simulink model "CP_DTSFC_Lin_b_9558292"  (R2018a)
settings: Solver=FixedStepDiscrete  StartTime=0.0  StopTime=3  FixedStep=T_s  RelTol=1e-3
values from neighbouring files (symbols this model uses):
  K_db = place(sysdzoh.A,sysdzoh.B,Pb_d)    [CP_DTSFC_Lin_b_MainFile_9558292.m]
  sysdzoh = c2d(sysc,T_s,'zoh')    [CP_DTSFC_Lin_a_MainFile_n9558292.m]    (also in CP_DTSFC_Lin_b_MainFile_9558292.m)
  T_s = 0.03    [CP_DTSFC_Lin_a_MainFile_n9558292.m]    (also in CP_DTSFC_Lin_b_MainFile_9558292.m)
  x10 = 0.2    [CP_DTSFC_Lin_a_MainFile_n9558292.m]    (also in CP_DTSFC_Lin_b_MainFile_9558292.m)
  x20 = deg2rad(20)    [CP_DTSFC_Lin_a_MainFile_n9558292.m]    (also in CP_DTSFC_Lin_b_MainFile_9558292.m)
  x30 = 0    [CP_DTSFC_Lin_a_MainFile_n9558292.m]    (also in CP_DTSFC_Lin_b_MainFile_9558292.m)
  x40 = 0    [CP_DTSFC_Lin_a_MainFile_n9558292.m]    (also in CP_DTSFC_Lin_b_MainFile_9558292.m)
settings Model: Creator=haidarobeid  LastModifiedBy=haidarobeid

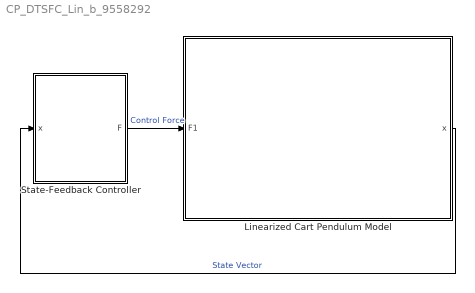
== system CP_DTSFC_Lin_b_9558292 ==
  Linearized Cart Pendulum Model : Subsystem
  State-Feedback Controller : Subsystem
  wires:
  Linearized Cart Pendulum Model/1(x) -> State-Feedback Controller/1(x)  "State Vector"
  State-Feedback Controller/1(F) -> Linearized Cart Pendulum Model/1(F1)  "Control Force"

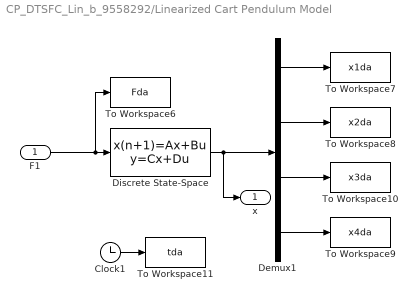
== system CP_DTSFC_Lin_b_9558292/Linearized Cart Pendulum Model ==
  F1 : Inport
  Clock1 : Clock
  Demux1 : Demux
  Discrete State-Space : DiscreteStateSpace  A=sysdzoh.A  B=sysdzoh.B  C=sysdzoh.C  D=sysdzoh.D  InitialCondition=[x10;x20;x30;x40]  SampleTime=T_s
  To Workspace10 : ToWorkspace  VariableName=x3da  SampleTime=-1
  To Workspace11 : ToWorkspace  VariableName=tda  SampleTime=-1
  To Workspace6 : ToWorkspace  VariableName=Fda  SampleTime=-1
  To Workspace7 : ToWorkspace  VariableName=x1da  SampleTime=-1
  To Workspace8 : ToWorkspace  VariableName=x2da  SampleTime=-1
  To Workspace9 : ToWorkspace  VariableName=x4da  SampleTime=-1
  x : Outport
  wires:
  Demux1/4 -> To Workspace9/1
  Discrete State-Space/1 -> Demux1/1, x/1
  F1/1 -> To Workspace6/1, Discrete State-Space/1
  Demux1/3 -> To Workspace10/1
  Demux1/2 -> To Workspace8/1
  Demux1/1 -> To Workspace7/1
  Clock1/1 -> To Workspace11/1

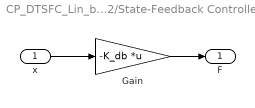
== system CP_DTSFC_Lin_b_9558292/State-Feedback Controller ==
  x : Inport
  Gain : Gain  Gain=-K_db  Multiplication=Matrix(K*u)
  F : Outport
  wires:
  Gain/1 -> F/1
  x/1 -> Gain/1
